simulink model "BMS_Harness_fullBMS"  (R2025b)
settings: configuration reference "AutosarConfig" (kept outside this file)
undefined symbols (not defined in the file): cellVoltBasic, StateReq
libraries: SignalEditorBlockLib x1
settings Model: DataDictionary=BMS_Software_DD.sldd  Creator=smuckati  LastModifiedBy=smuckati
settings ConfigSetRef: SourceName=AutosarConfig

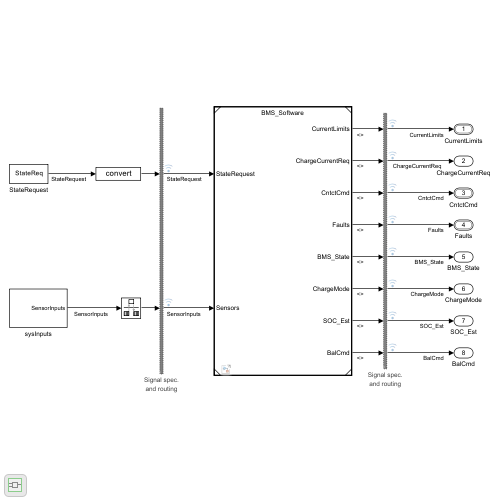
[thumbnail: Simulink's stored preview of the top-level diagram]
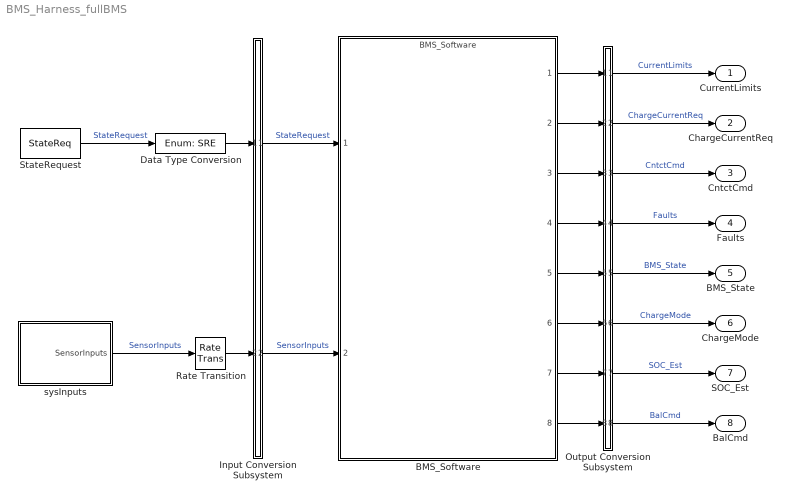
== system BMS_Harness_fullBMS ==
  BMS_Software : ModelReference  ModelNameDialog=BMS_Software  SimulationMode=Normal  ModelReferenceVersion=11.4
  Data Type Conversion : DataTypeConversion  OutDataTypeStr=Enum: SRE  SaturateOnIntegerOverflow=off  RndMeth=Floor
  Input Conversion Subsystem : Subsystem  Tag=__SLT_ICS__  Description=|
      | Signal spec.
      | and routing
      settings: AttributesFormatString=%<Description>
  Output Conversion Subsystem : Subsystem  Tag=__SLT_OCS__  Description=|
      | Signal spec.
      | and routing
      settings: AttributesFormatString=%<Description>
  Rate Transition : RateTransition  OutPortSampleTime=0.1
  StateRequest : Constant  Value=StateReq  OutDataTypeStr=int8
  sysInputs : Subsystem
  CurrentLimits : Outport  OutDataTypeStr=Bus: CurrentLimits
  ChargeCurrentReq : Outport  Port=2
  CntctCmd : Outport  Port=3  OutDataTypeStr=Bus: CntctCmd
  Faults : Outport  Port=4  OutDataTypeStr=Bus: Faults
  BMS_State : Outport  Port=5
  ChargeMode : Outport  Port=6
  SOC_Est : Outport  Port=7
  BalCmd : Outport  Port=8
  wires:
  StateRequest/1 -> Data Type Conversion/1  "StateRequest"
  sysInputs/1(SensorInputs) -> Rate Transition/1  "SensorInputs"
  Output Conversion Subsystem/1(Outport_1) -> CurrentLimits/1  "CurrentLimits"
  Output Conversion Subsystem/2(Outport_2) -> ChargeCurrentReq/1  "ChargeCurrentReq"
  Output Conversion Subsystem/3(Outport_3) -> CntctCmd/1  "CntctCmd"
  Output Conversion Subsystem/4(Outport_4) -> Faults/1  "Faults"
  Output Conversion Subsystem/5(Outport_5) -> BMS_State/1  "BMS_State"
  Output Conversion Subsystem/6(Outport_6) -> ChargeMode/1  "ChargeMode"
  Output Conversion Subsystem/7(Outport_7) -> SOC_Est/1  "SOC_Est"
  Output Conversion Subsystem/8(Outport_8) -> BalCmd/1  "BalCmd"
  Input Conversion Subsystem/1(Outport_1) -> BMS_Software/1  "StateRequest"
  Input Conversion Subsystem/2(Outport_2) -> BMS_Software/2  "SensorInputs"
  BMS_Software/1 -> Output Conversion Subsystem/1(Inport_1)
  BMS_Software/2 -> Output Conversion Subsystem/2(Inport_2)
  BMS_Software/3 -> Output Conversion Subsystem/3(Inport_3)
  BMS_Software/4 -> Output Conversion Subsystem/4(Inport_4)
  BMS_Software/5 -> Output Conversion Subsystem/5(Inport_5)
  BMS_Software/6 -> Output Conversion Subsystem/6(Inport_6)
  BMS_Software/7 -> Output Conversion Subsystem/7(Inport_7)
  BMS_Software/8 -> Output Conversion Subsystem/8(Inport_8)
  Rate Transition/1 -> Input Conversion Subsystem/2(Inport_2)
  Data Type Conversion/1 -> Input Conversion Subsystem/1(Inport_1)

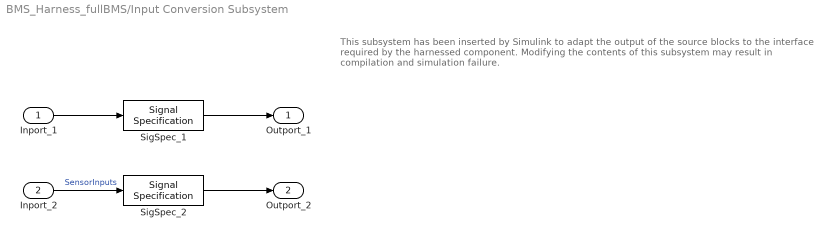
== system BMS_Harness_fullBMS/Input Conversion Subsystem ==
  note: This subsystem has been inserted by Simulink to adapt the output of the source blocks to the interface required by the harnessed component.
      |  Modifying the contents of this subsystem may result in compilation and simulation failure.
  Inport_1 : Inport
  Inport_2 : Inport  Port=2
  SigSpec_1 : SignalSpecification  OutDataTypeStr=Enum: SRE  Dimensions=[1]  SampleTime=0.1
  SigSpec_2 : SignalSpecification  OutDataTypeStr=Bus: Sensors  Dimensions=[1]  SampleTime=0.1  BusOutputAsStruct=on
  Outport_1 : Outport
  Outport_2 : Outport  Port=2
  wires:
  SigSpec_1/1 -> Outport_1/1
  Inport_1/1 -> SigSpec_1/1
  SigSpec_2/1 -> Outport_2/1
  Inport_2/1 -> SigSpec_2/1  "SensorInputs"

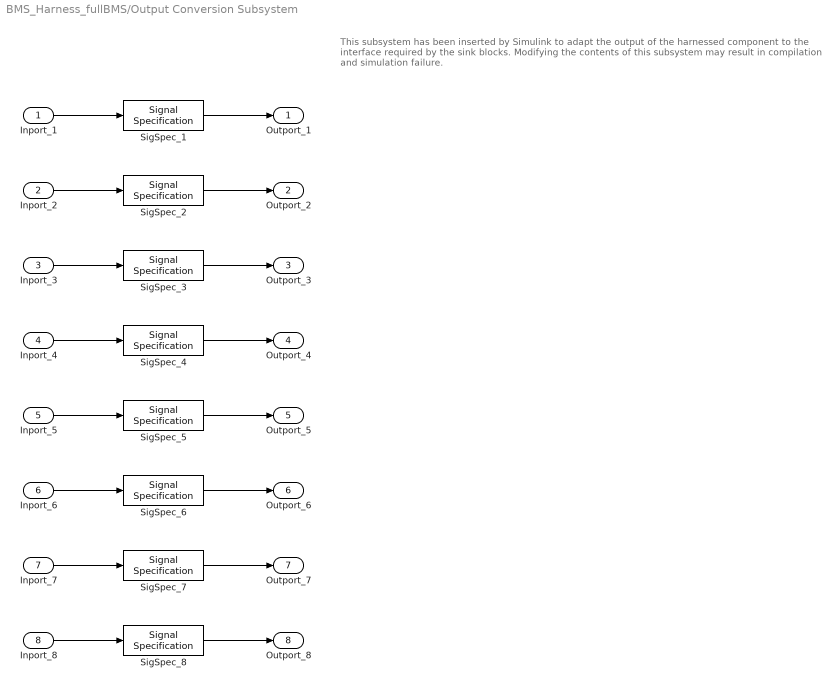
== system BMS_Harness_fullBMS/Output Conversion Subsystem ==
  note: This subsystem has been inserted by Simulink to adapt the output of the harnessed component to the interface required by the sink blocks.
      |  Modifying the contents of this subsystem may result in compilation and simulation failure.
  Inport_1 : Inport
  Inport_2 : Inport  Port=2
  Inport_3 : Inport  Port=3
  Inport_4 : Inport  Port=4
  Inport_5 : Inport  Port=5
  Inport_6 : Inport  Port=6
  Inport_7 : Inport  Port=7
  Inport_8 : Inport  Port=8
  SigSpec_1 : SignalSpecification  OutDataTypeStr=Bus: CurrentLimits  Dimensions=[1]  SampleTime=0.1
  SigSpec_2 : SignalSpecification  OutDataTypeStr=single  Dimensions=[1]  SampleTime=0.1
  SigSpec_3 : SignalSpecification  OutDataTypeStr=Bus: CntctCmd  Dimensions=[1]  SampleTime=0.1
  SigSpec_4 : SignalSpecification  OutDataTypeStr=Bus: Faults  Dimensions=[1]  SampleTime=0.1
  SigSpec_5 : SignalSpecification  OutDataTypeStr=Enum: BMS_State_Enum  Dimensions=[1]  SampleTime=0.1
  SigSpec_6 : SignalSpecification  OutDataTypeStr=Enum: ChargeMode_Enum  Dimensions=[1]  SampleTime=0.1
  SigSpec_7 : SignalSpecification  OutDataTypeStr=single  Dimensions=[1]  SampleTime=0.1
  SigSpec_8 : SignalSpecification  OutDataTypeStr=boolean  Dimensions=[1, 96]  SampleTime=0.1
  Outport_1 : Outport
  Outport_2 : Outport  Port=2
  Outport_3 : Outport  Port=3
  Outport_4 : Outport  Port=4
  Outport_5 : Outport  Port=5
  Outport_6 : Outport  Port=6
  Outport_7 : Outport  Port=7
  Outport_8 : Outport  Port=8
  wires:
  Inport_1/1 -> SigSpec_1/1
  SigSpec_1/1 -> Outport_1/1
  Inport_2/1 -> SigSpec_2/1
  SigSpec_2/1 -> Outport_2/1
  Inport_3/1 -> SigSpec_3/1
  SigSpec_3/1 -> Outport_3/1
  Inport_4/1 -> SigSpec_4/1
  SigSpec_4/1 -> Outport_4/1
  Inport_5/1 -> SigSpec_5/1
  SigSpec_5/1 -> Outport_5/1
  Inport_6/1 -> SigSpec_6/1
  SigSpec_6/1 -> Outport_6/1
  Inport_7/1 -> SigSpec_7/1
  SigSpec_7/1 -> Outport_7/1
  Inport_8/1 -> SigSpec_8/1
  SigSpec_8/1 -> Outport_8/1

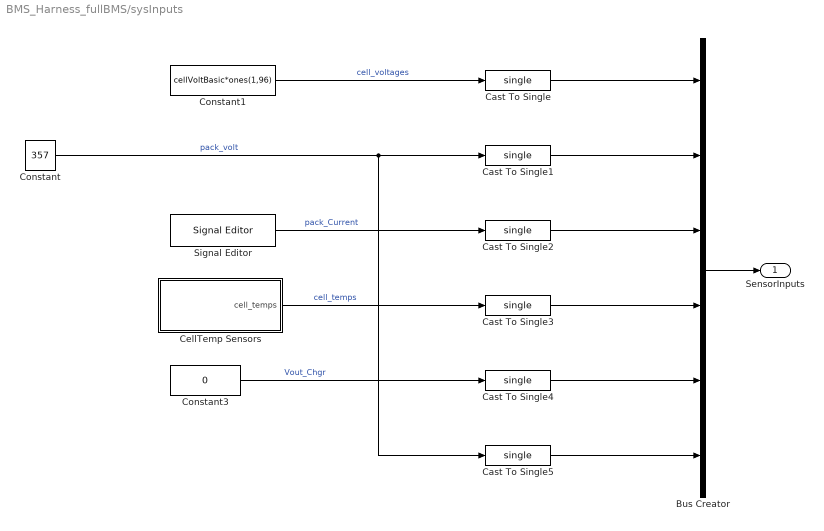
== system BMS_Harness_fullBMS/sysInputs ==
  Bus Creator : BusCreator  Inputs=6  OutDataTypeStr=Bus: Sensors  NonVirtualBus=on
      settings: InheritFromInputs=off
  Cast To Single{,1..5} (6 alike) : DataTypeConversion  OutDataTypeStr=single  SaturateOnIntegerOverflow=off  RndMeth=Floor
  CellTemp Sensors : Subsystem
  Constant : Constant  Value=357
  Constant1 : Constant  Value=cellVoltBasic*ones(1,96)
  Constant3 : Constant  Value=0
  Signal Editor : SignalEditorBlockLib/Signal Editor  FileName=PowerCalc_HarnessInputs.mat  ActiveScenario=Scenario  ActiveSignal=PackCurrent  IsBus=off  OutputBusObjectStr=Bus: BusObject  SampleTime=0  Interpolate=off  ZeroCross=off  OutputAfterFinalValue=Setting to zero  Unit=inherit  PreserveSignalName=on  ApplySigPropsToAllScenarios=on  ApplySigPropsToAllSignals=off  SignalPropertySource=Dialog parameters
  SensorInputs : Outport
  wires:
  Bus Creator/1 -> SensorInputs/1
  Constant1/1 -> Cast To Single/1  "cell_voltages"
  Constant/1 -> Cast To Single5/1, Cast To Single1/1  "pack_volt"
  CellTemp Sensors/1(cell_temps) -> Cast To Single3/1  "cell_temps"
  Constant3/1 -> Cast To Single4/1  "Vout_Chgr"
  Signal Editor/1 -> Cast To Single2/1  "pack_Current"
  Cast To Single/1 -> Bus Creator/1
  Cast To Single1/1 -> Bus Creator/2
  Cast To Single2/1 -> Bus Creator/3
  Cast To Single3/1 -> Bus Creator/4
  Cast To Single4/1 -> Bus Creator/5
  Cast To Single5/1 -> Bus Creator/6

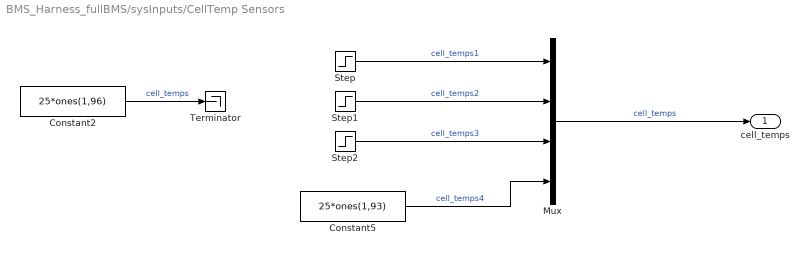
== system BMS_Harness_fullBMS/sysInputs/CellTemp Sensors ==
  Constant2 : Constant  Value=25*ones(1,96)
  Constant5 : Constant  Value=25*ones(1,93)
  Mux : Mux
  Step : Step  Time=400  Before=24  After=14  SampleTime=0
      settings: AttributesFormatString=Tfinal = 14
  Step1 : Step  Time=400  Before=24  After=14  SampleTime=0
      settings: AttributesFormatString=Tfinal = 14
  Step2 : Step  Time=400  Before=24  After=12  SampleTime=0
      settings: AttributesFormatString=Tfinal = 12
  Terminator : Terminator
  cell_temps : Outport
  wires:
  Constant5/1 -> Mux/4  "cell_temps4"
  Constant2/1 -> Terminator/1  "cell_temps"
  Step1/1 -> Mux/2  "cell_temps2"
  Mux/1 -> cell_temps/1  "cell_temps"
  Step/1 -> Mux/1  "cell_temps1"
  Step2/1 -> Mux/3  "cell_temps3"
